simulink model "MLIB_Abs_BAM"  (Simulink 7.3)
settings: Solver=ode45  StartTime=0.0  StopTime=10.0  RelTol=1e-3
settings Model: Creator=RE004C  LastModifiedBy=RE004C
settings HardwareCC: ProdIntDivRoundTo=Zero  ProdEndianess=BigEndian  ProdHWDeviceType=Freescale->32-bit PowerPC

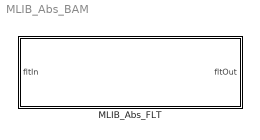
== system MLIB_Abs_BAM ==
  MLIB_Abs_FLT : Subsystem  mask(MLIB_Abs_FLT){}
      mask help: Bit accurate model for absolute value of input value. All parameters as well as input and output are 32bit integers.
      mask init:
      | pos = get_param(gcb, 'Position');width = pos(3) - pos(1); height = pos(4) - pos(2);tX=width/2;tY=height*0.9;
      mask Display: color('black');port_label('input',1,'fltIn');port_label('output',1,'fltOut');color('black');disp('MLIB_Abs_FLT');color('blue');text(tX,tY, 'BAM', 'horizontalAlignment', 'center');

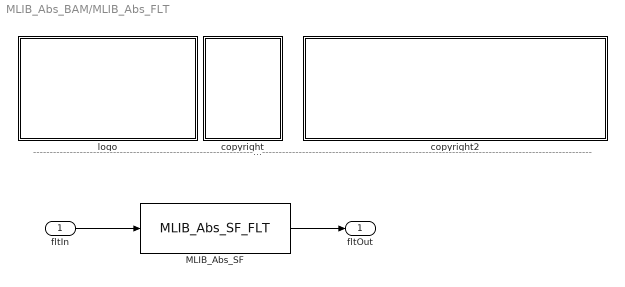
== system MLIB_Abs_BAM/MLIB_Abs_FLT ==
  note: ---------------------------------------------------------------------------------------------------------------------------------------------------------------------------------------------------
  fltIn : Inport  OutDataType=fixdt(1, 16)  OutScaling=2^0
  MLIB_Abs_SF : S-Function  FunctionName=MLIB_Abs_SF_FLT  EnableBusSupport=off
  copyright : Subsystem
      mask Display: text(10,90,'FILE:');text(10,75,'DESRIPTION:')text(10,60,'COPYRIGHT:')text(10,45,'VERSION:')text(10,30,'DATE:')
  copyright2 : Subsystem
      mask Display: text(10,90,'MLIB_Abs_BAM_FLT.mdl');text(10,75,'Absolute value of input parameter.');text(10,60,'Freescale')text(10,45,'0.1');text(10,30,'20-Jan-2012');
  logo : Subsystem
      mask Display: image(imread('logo.jpg'))
  fltOut : Outport  OutDataType=fixdt(1, 16)  OutScaling=2^0
  wires:
  fltIn/1 -> MLIB_Abs_SF/1
  MLIB_Abs_SF/1 -> fltOut/1

== system MLIB_Abs_BAM/MLIB_Abs_FLT/copyright ==

== system MLIB_Abs_BAM/MLIB_Abs_FLT/copyright2 ==

== system MLIB_Abs_BAM/MLIB_Abs_FLT/logo ==
